simulink model "pmsm"  (R2024a)
settings: Solver=FixedStepAuto  StartTime=0.0  StopTime=5  FixedStep=1e-3  RelTol=1e-3
libraries: spsControlledVoltageSourceLib x6, simulink x6, spsGroundLib x2, ee_lib x1, spsPermanentMagnetSynchronousMachineLib x1, spsThreePhaseSeriesRLCBranchLib x1, spsThreePhaseVIMeasurementLib x1, sps_lib x1
settings Model: Creator=ammarabdulrasheed  LastModifiedBy=ammarabdulrasheed

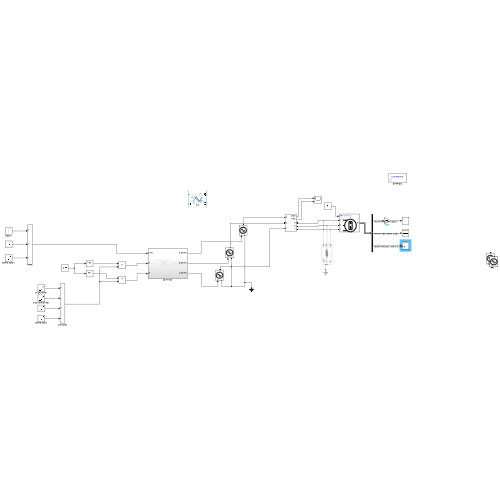
[thumbnail: Simulink's stored preview of the top-level diagram]
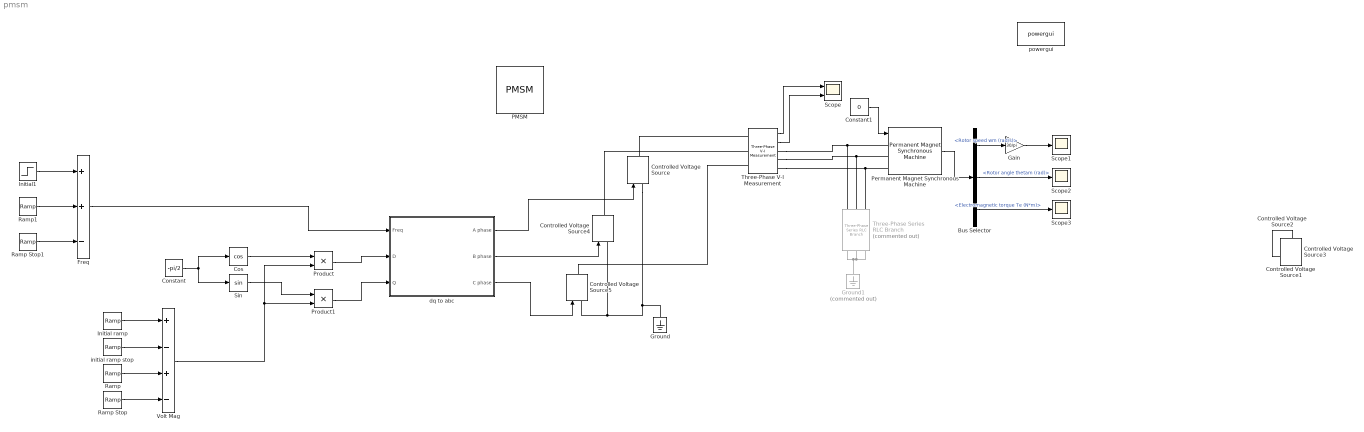
== system pmsm ==
  Bus Selector : BusSelector  OutputSignals=Rotor speed wm (rad/s),Rotor angle thetam (rad),Electromagnetic torque Te (N*m)
  Constant : Constant  Value=-pi/2
  Constant1 : Constant  Value=0
  Controlled Voltage Source{,1..5} (6 alike) : spsControlledVoltageSourceLib/Controlled Voltage Source  Initialize=on  Source_Type=AC  Amplitude=0  Phase=0  Frequency=0  Measurements=None
  Cos : Trigonometry  Operator=cos
  Freq : Sum  Inputs=++-
  Gain : Gain  Gain=30/pi
  Ground : spsGroundLib/Ground  LConnTagsString=a
  Ground1 : spsGroundLib/Ground  Commented=on  LConnTagsString=a
  Initial ramp : simulink/Sources/Ramp  slope=10  start=0  InitialOutput=0
  Initial1 : Step  Time=0  After=0  SampleTime=0
  PMSM : ee_lib/Electromechanical/Permanent Magnet/PMSM  port_option=ee.enum.threePhasePort.composite  winding_type=ee.enum.electromech.statorconfiguration.wye  machine_param=ee.enum.pmsm.parameterization.constant  nPolePairs=6  pmflux_param=ee.enum.pmflux.fluxlinkage  pm_flux_linkage=0.03 Wb  torque_constant=0.18 N*m/A  back_emf_constant=0.18 V*s/rad  stator_param=ee.enum.statorparam.LdLqL0  Ld=0.00019 H  Lq=0.00025 H  idVec=[-200, 0, 200] A  iqVec=[-200, 0, 200] A  LdMatrix=0.0002 * ones(3, 3) H  LqMatrix=0.0002 * ones(3, 3) H  PmMatrix=0.1 * ones(3, 3) Wb  ktMatrix=0.18 * ones(3, 3) N*m/A  keMatrix=0.18 * ones(3, 3) V*s/rad  L0=0.00016 H  Ls=0.0002 H  Lm=-0.00002 H  Ms=0.00002 H  Rs=0.013 Ohm  zero_sequence=ee.enum.park.zerosequence.include  axes_param=ee.enum.rotorangle.daxis  loss_param=ee.enum.ironloss.none  losses_oc=[0, 0, 0] W  losses_sc=[0, 0, 0] W  f_losses=60 Hz  Isc_losses=95 A  J=0.01 kg*m^2  lam=0 N*m*s/rad  i_d_specify=off  i_d_priority=None  i_d=0 A  i_d_nominal_specify=off  i_d_nominal_value=1  i_d_nominal_unit=A  i_q_specify=off  i_q_priority=None  i_q=0 A  i_q_nominal_specify=off  i_q_nominal_value=1  i_q_nominal_unit=A  torque_specify=off  torque_priority=None  torque=0 N*m  torque_nominal_specify=off  torque_nominal_value=1  torque_nominal_unit=N*m  angular_velocity_specify=off  angular_velocity_priority=High  angular_velocity=0 rpm  angular_velocity_nominal_specify=off  angular_velocity_nominal_value=1  angular_velocity_nominal_unit=rpm  angular_position_specify=off  angular_position_priority=High  angular_position=0 deg  angular_position_nominal_specify=off  angular_position_nominal_value=1  angular_position_nominal_unit=deg  alpha=3.93e-3 1/K  alpha_flux=-0.001 1/K  Tmeas=298.15 K  stator_thermal_mass=100 J/K  rotor_thermal_mass=200 J/K  Rm_percent_rotor=90  Rd_percent_rotor=30  temperatureA_specify=off  temperatureA_priority=High  temperatureA=25 degC  temperatureA_nominal_specify=off  temperatureA_nominal_value=1  temperatureA_nominal_unit=degC  temperatureB_specify=off  temperatureB_priority=High  temperatureB=25 degC  temperatureB_nominal_specify=off  temperatureB_nominal_value=1  temperatureB_nominal_unit=degC  temperatureC_specify=off  temperatureC_priority=High  temperatureC=25 degC  temperatureC_nominal_specify=off  temperatureC_nominal_value=1  temperatureC_nominal_unit=degC  temperatureR_specify=off  temperatureR_priority=High  temperatureR=25 degC  temperatureR_nominal_specify=off  temperatureR_nominal_value=1  temperatureR_nominal_unit=degC
      settings: InternalSimscapePortConfiguration="{\"Bottom\":[],\"Left\":[{\"id\":\"N\",\"label\":\"~\",\"type\":\"foundation.electrical.three_phase\"},{\"id\":\"n\",\"label\":\"n\",\"type\":\"foundation.electrical.electrical\"}],\"Right\":[{\"id\":\"R\",\"label\":\"R\",\"type\":\"foundation.mechanical.rotational.rotational\"},{\"id\":\"C\",\"label\":\"C\",\"type\":\"foundation.mechanical.rotational.rotational\"}],\"Top\":[]}"
  Permanent Magnet Synchronous Machine : spsPermanentMagnetSynchronousMachineLib/Permanent Magnet Synchronous Machine  NbPhases=3  FluxDistribution=Sinusoidal  RotorType=Round  MechanicalLoad=Torque Tm  PresetModel=No  ShowDetailedParameters=on  MeasurementBus=off  Resistance=1.93  Inductance=8.5e-3  dqInductances=[8.5e-3,8.5e-3]  La=92.19e-3  MachineConstant=Flux linkage established by magnets (V.s)  Flux=0.311  VoltageCst=112.8183  TorqueCst=0.933  Flat=120  Mechanical=[0.003 0.001 2 0]  PolePairs=4  InitialConditions=[0,0, 0,0]  InitialConditions5ph=[0 0 0 0 0 0]  RefAngle=90 degrees behind phase A axis (modified Park)  IterativeDiscreteModel=Trapezoidal non iterative  TsBlock=-1  TsPowergui=0
  Product : Product
  Product1 : Product
  Ramp : simulink/Sources/Ramp  slope=25*4  start=1 + 5/(4*25)  InitialOutput=0
  Ramp Stop : simulink/Sources/Ramp  slope=25*4  start=3  InitialOutput=0
  Ramp Stop1 : simulink/Sources/Ramp  slope=25  start=3  InitialOutput=0
  Ramp1 : simulink/Sources/Ramp  slope=25  start=1  InitialOutput=0
  Scope : Scope  NumInputPorts=2
  Scope1 : Scope
  Scope2 : Scope
  Scope3 : Scope
  Sin : Trigonometry
  Three-Phase Series RLC Branch : spsThreePhaseSeriesRLCBranchLib/Three-Phase Series RLC Branch  Commented=on  LConnTagsString=A|B|C  RConnTagsString=A|B|C  BranchType=R  Resistance=1e3  Inductance=1e-3  Capacitance=1e-6  Measurements=None
  Three-Phase V-I Measurement : spsThreePhaseVIMeasurementLib/Three-Phase V-I Measurement  VoltageMeasurement=phase-to-ground  SetLabelV=off  LabelV=Vabc  Vpu=off  VpuLL=off  CurrentMeasurement=yes  SetLabelI=off  LabelI=Iabc  Ipu=off  Pbase=100e6  Vbase=500e3  OutputType=Complex  PhasorSimulation=off  PSBequivalent=0
  Volt Mag : Sum  Inputs=+-+-
  dq to abc : Subsystem
  initial ramp stop : simulink/Sources/Ramp  slope=10  start=0.5  InitialOutput=0
  powergui : sps_lib/powergui  Priority=1  SimulationMode=Continuous  SampleTime=50e-6  frequency=60  Iterations=50  frequencyindice=0  Pbase=100e6  ErrMax=1e-4  UnitsV=kV  UnitsW=MW  buscounter=0  FunctionMessages=off  echomessages=off  EnableUseOfTLC=off  CurrentSourceSwitches=off  DisableSnubberDevices=off  DisableRonSwitches=off  DisableVfSwitches=off  DisplayEquations=off  AutomaticDiscreteSolvers=off  SolverType=Tustin/Backward Euler (TBE)  Interpol=off  ExternalGateDelay=off  methode=off  Ts=100  x0status=blocks  SPID=on  SwTol=0  HookPort=off  NonlinearTolerance=1e-4  nMaxIteration=100  ContinueOnMaxIteration=off  RestoreLinks=warning  ResistiveCurrentMeasurement=off  Frange=[0:2:500]  Ylog=off  Xlog=on  ShowGrid=off  save=off  variable=ZData  structure=0  ZoomFFT=off  StartTime=0.0  cycles=1  DisplayStyle=1  fundamental=60  FreqAxis=off  MaxFrequency=1000  frequencyindicesteady=1  RmsSteady=1  display=off
  wires:
  Ramp Stop1/1 -> Freq/3
  Initial1/1 -> Freq/1
  Ramp1/1 -> Freq/2
  Freq/1 -> dq to abc/1(Freq)
  Constant/1 -> Sin/1, Cos/1
  dq to abc/1(A phase) -> Controlled Voltage Source/1
  dq to abc/2(B phase) -> Controlled Voltage Source4/1
  dq to abc/3(C phase) -> Controlled Voltage Source5/1
  Three-Phase V-I Measurement/1 -> Scope/1
  Constant1/1 -> Permanent Magnet Synchronous Machine/1
  Permanent Magnet Synchronous Machine/1 -> Bus Selector/1
  Bus Selector/1 -> Gain/1  "<Rotor speed wm (rad/s)>"
  Cos/1 -> Product/1
  Product/1 -> dq to abc/2(D)
  Sin/1 -> Product1/1
  Product1/1 -> dq to abc/3(Q)
  Ramp Stop/1 -> Volt Mag/4
  Ramp/1 -> Volt Mag/3
  Initial ramp/1 -> Volt Mag/1
  initial ramp stop/1 -> Volt Mag/2
  Volt Mag/1 -> Product1/2, Product/2
  Three-Phase V-I Measurement/2 -> Scope/2
  Gain/1 -> Scope1/1
  Bus Selector/2 -> Scope2/1  "<Rotor angle thetam (rad)>"
  Bus Selector/3 -> Scope3/1  "<Electromagnetic torque Te (N*m)>"
  connections:
  Controlled Voltage Source/LConn1 -- Ground/LConn1 -- Controlled Voltage Source5/LConn1 -- Controlled Voltage Source4/LConn1
  Controlled Voltage Source/RConn1 -- Three-Phase V-I Measurement/LConn1
  Controlled Voltage Source4/RConn1 -- Three-Phase V-I Measurement/LConn2
  Controlled Voltage Source5/RConn1 -- Three-Phase V-I Measurement/LConn3
  Three-Phase V-I Measurement/RConn1 -- Three-Phase Series RLC Branch/LConn1 -- Permanent Magnet Synchronous Machine/LConn1
  Three-Phase V-I Measurement/RConn2 -- Three-Phase Series RLC Branch/LConn2 -- Permanent Magnet Synchronous Machine/LConn2
  Three-Phase V-I Measurement/RConn3 -- Three-Phase Series RLC Branch/LConn3 -- Permanent Magnet Synchronous Machine/LConn3
  Three-Phase Series RLC Branch/RConn1 -- Three-Phase Series RLC Branch/RConn2 -- Three-Phase Series RLC Branch/RConn3 -- Ground1/LConn1

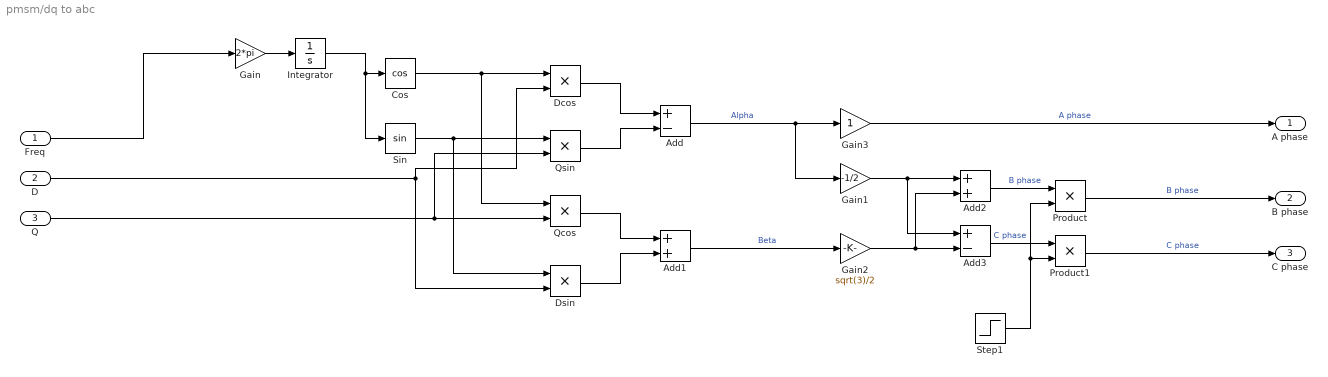
== system pmsm/dq to abc ==
  Freq : Inport
  D : Inport  Port=2
  Q : Inport  Port=3
  Add : Sum  Inputs=+-
  Add1 : Sum
  Add2 : Sum
  Add3 : Sum  Inputs=+-
  Cos : Trigonometry  Operator=cos
  Dcos : Product
  Dsin : Product
  Gain : Gain  Gain=2*pi
  Gain1 : Gain  Gain=-1/2
  Gain2 : Gain  Gain=sqrt(3)/2
  Gain3 : Gain
  Integrator : Integrator
  Product : Product
  Product1 : Product
  Qcos : Product
  Qsin : Product
  Sin : Trigonometry
  Step1 : Step  Time=0  SampleTime=0
  A phase : Outport
  B phase : Outport  Port=2
  C phase : Outport  Port=3
  wires:
  Product/1 -> B phase/1  "B phase"
  Add1/1 -> Gain2/1  "Beta"
  Product1/1 -> C phase/1  "C phase"
  D/1 -> Dsin/2, Dcos/2
  Dsin/1 -> Add1/2
  Freq/1 -> Gain/1
  Step1/1 -> Product1/2, Product/2
  Q/1 -> Qcos/2, Qsin/2
  Dcos/1 -> Add/1
  Gain/1 -> Integrator/1
  Gain3/1 -> A phase/1  "A phase"
  Cos/1 -> Qcos/1, Dcos/1
  Add2/1 -> Product/1  "B phase"
  Gain2/1 -> Add3/2, Add2/2
  Integrator/1 -> Sin/1, Cos/1
  Add3/1 -> Product1/1  "C phase"
  Sin/1 -> Dsin/1, Qsin/1
  Gain1/1 -> Add3/1, Add2/1
  Qsin/1 -> Add/2
  Qcos/1 -> Add1/1
  Add/1 -> Gain1/1, Gain3/1  "Alpha"
